simulink model "abslut50_fixpt8_19"  (R2021b)
settings: Solver=VariableStepAuto  StartTime=0.0  StopTime=99  RelTol=1e-3
undefined symbols (not defined in the file or in its folder): figd2104, xcu250
libraries: hdlBasic x4666, vmcUtilities x1
(part 1 of 15)
settings Model: Creator=shu_abe  LastModifiedBy=shu_abe

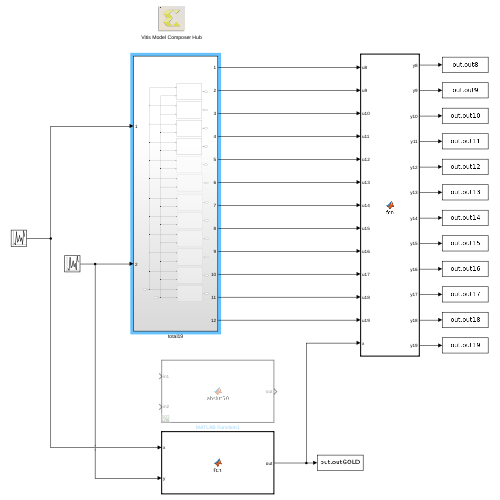
[thumbnail: Simulink's stored preview of the top-level diagram]
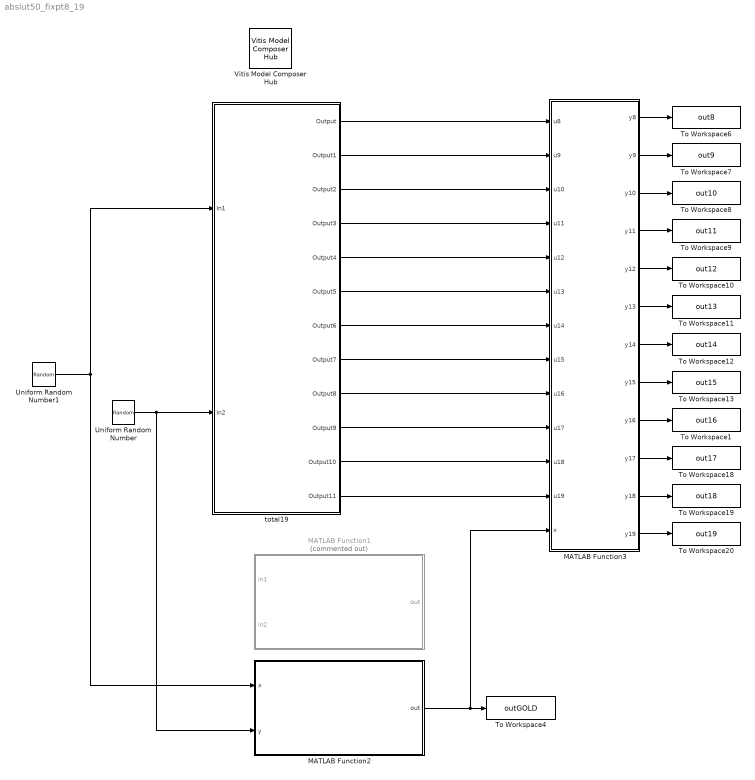
== system abslut50_fixpt8_19 ==
  MATLAB Function1 : MATLAB Function  Commented=on  TreatAsAtomicUnit=on
  MATLAB Function2 : MATLAB Function  TreatAsAtomicUnit=on
  MATLAB Function3 : MATLAB Function  TreatAsAtomicUnit=on
  To Workspace1 : ToWorkspace  VariableName=out16  SaveFormat=Structure With Time  SampleTime=-1
  To Workspace10 : ToWorkspace  VariableName=out12  SaveFormat=Structure With Time  SampleTime=-1
  To Workspace11 : ToWorkspace  VariableName=out13  SaveFormat=Structure With Time  SampleTime=-1
  To Workspace12 : ToWorkspace  VariableName=out14  SaveFormat=Structure With Time  SampleTime=-1
  To Workspace13 : ToWorkspace  VariableName=out15  SaveFormat=Structure With Time  SampleTime=-1
  To Workspace18 : ToWorkspace  VariableName=out17  SaveFormat=Structure With Time  SampleTime=-1
  To Workspace19 : ToWorkspace  VariableName=out18  SaveFormat=Structure With Time  SampleTime=-1
  To Workspace20 : ToWorkspace  VariableName=out19  SaveFormat=Structure With Time  SampleTime=-1
  To Workspace4 : ToWorkspace  VariableName=outGOLD  SaveFormat=Structure With Time  SampleTime=1
  To Workspace6 : ToWorkspace  VariableName=out8  SaveFormat=Structure With Time  SampleTime=-1
  To Workspace7 : ToWorkspace  VariableName=out9  SaveFormat=Structure With Time  SampleTime=-1
  To Workspace8 : ToWorkspace  VariableName=out10  SaveFormat=Structure With Time  SampleTime=-1
  To Workspace9 : ToWorkspace  VariableName=out11  SaveFormat=Structure With Time  SampleTime=-1
  Uniform Random Number : UniformRandomNumber  Minimum=-0.9  Maximum=0.9  SampleTime=1
  Uniform Random Number1 : UniformRandomNumber  Minimum=-0.9  Maximum=0.9  Seed=1  SampleTime=1
  Vitis Model Composer Hub : vmcUtilities/Vitis Model Composer Hub  Tag=genX  CodeGeneration=off  SubsystemName=<enter or select subsystem name>  TargetDirectory=./code  ExportType=HLS C++ code  IpVendor=xilinx.com  IpLibrary=hls  IpVersion=1.0  IpHWLanguage=Verilog  AieCompilerOptions={}  CreateTestbench=off  TestbenchStackSize=10  RunAieSim=off  AieSimTimeout=50000  RunAieSimProfiling=off  LaunchVitisAnalyzer=off  PlotOutput=off  RunX86Sim=off  X86SimTimeout=10  GenHwImage=off  PlatformType=Not Specified  HwSystemType=Baremetal  HwValidationTarget=hw  ProjDevice=Alveo U250 Data Center Accelerator Card (xcu250-figd2104-2L-e)  ProjDevicePart=xcu250-figd2104-2L-e  SamplePeriod=-1  ClockFrequency=200  DataPathParallelism=1  xilinxfamily=virtexuplus  part=xcu250  speed=-2L-e  package=figd2104  directory=./abslut50_fixpt19  testbench=off  incr_netlist=off  synthesis_tool=Vivado  clock_wrapper=Clock Enables  dbl_ovrd=According to Block Masks  dcm_input_clock_period=10  sysclk_period=50  simulink_period=1  eval_field=0
  total19 : Subsystem
  wires:
  MATLAB Function2/1(out) -> MATLAB Function3/13(x), To Workspace4/1
  Uniform Random Number1/1 -> MATLAB Function2/1(x), total19/1(In1)
  Uniform Random Number/1 -> MATLAB Function2/2(y), total19/2(In2)
  MATLAB Function3/1(y8) -> To Workspace6/1
  MATLAB Function3/4(y11) -> To Workspace9/1
  MATLAB Function3/2(y9) -> To Workspace7/1
  MATLAB Function3/12(y19) -> To Workspace20/1
  MATLAB Function3/3(y10) -> To Workspace8/1
  MATLAB Function3/9(y16) -> To Workspace1/1
  MATLAB Function3/8(y15) -> To Workspace13/1
  MATLAB Function3/5(y12) -> To Workspace10/1
  MATLAB Function3/7(y14) -> To Workspace12/1
  MATLAB Function3/6(y13) -> To Workspace11/1
  MATLAB Function3/10(y17) -> To Workspace18/1
  MATLAB Function3/11(y18) -> To Workspace19/1
  total19/1(Output) -> MATLAB Function3/1(u8)
  total19/2(Output1) -> MATLAB Function3/2(u9)
  total19/3(Output2) -> MATLAB Function3/3(u10)
  total19/4(Output3) -> MATLAB Function3/4(u11)
  total19/5(Output4) -> MATLAB Function3/5(u12)
  total19/6(Output5) -> MATLAB Function3/6(u13)
  total19/7(Output6) -> MATLAB Function3/7(u14)
  total19/8(Output7) -> MATLAB Function3/8(u15)
  total19/9(Output8) -> MATLAB Function3/9(u16)
  total19/10(Output9) -> MATLAB Function3/10(u17)
  total19/11(Output10) -> MATLAB Function3/11(u18)
  total19/12(Output11) -> MATLAB Function3/12(u19)

== system abslut50_fixpt8_19/total19 ==
  In1 : Inport
  In2 : Inport  Port=2
  Subsystem10bit : Subsystem
  Subsystem11bit : Subsystem
  Subsystem12bit : Subsystem
  Subsystem13bit : Subsystem
  Subsystem14bit : Subsystem
  Subsystem15bit : Subsystem
  Subsystem16bit : Subsystem
  Subsystem17bit : Subsystem
  Subsystem18bit : Subsystem
  Subsystem19bit : Subsystem
  Subsystem8bit : Subsystem
  Subsystem9bit : Subsystem
  Output : Outport
  Output1 : Outport  Port=2
  Output2 : Outport  Port=3
  Output3 : Outport  Port=4
  Output4 : Outport  Port=5
  Output5 : Outport  Port=6
  Output6 : Outport  Port=7
  Output7 : Outport  Port=8
  Output8 : Outport  Port=9
  Output9 : Outport  Port=10
  Output10 : Outport  Port=11
  Output11 : Outport  Port=12
  wires:
  Subsystem12bit/1(Output) -> Output4/1
  Subsystem19bit/1(Output) -> Output11/1
  Subsystem10bit/1(Output) -> Output2/1
  Subsystem17bit/1(Output) -> Output9/1
  Subsystem16bit/1(Output) -> Output8/1
  In2/1 -> Subsystem16bit/2(In4), Subsystem15bit/2(In4), Subsystem14bit/2(In4), Subsystem13bit/2(In4), Subsystem12bit/2(In4), Subsystem10bit/2(In4), Subsystem8bit/2(In4), Subsystem9bit/2(In4), Subsystem11bit/2(In4), Subsystem17bit/2(In4), Subsystem18bit/2(In4), Subsystem19bit/2(In4)
  Subsystem18bit/1(Output) -> Output10/1
  Subsystem8bit/1(Output) -> Output/1
  Subsystem9bit/1(Output) -> Output1/1
  Subsystem11bit/1(Output) -> Output3/1
  In1/1 -> Subsystem17bit/1(In3), Subsystem15bit/1(In3), Subsystem13bit/1(In3), Subsystem12bit/1(In3), Subsystem11bit/1(In3), Subsystem10bit/1(In3), Subsystem8bit/1(In3), Subsystem9bit/1(In3), Subsystem14bit/1(In3), Subsystem16bit/1(In3), Subsystem18bit/1(In3), Subsystem19bit/1(In3)
  Subsystem13bit/1(Output) -> Output5/1
  Subsystem14bit/1(Output) -> Output6/1
  Subsystem15bit/1(Output) -> Output7/1
